simulink model "fuzzy_pid_control2"  (Simulink 8.7)
settings: Solver=VariableStepAuto  StartTime=0.0  StopTime=35  RelTol=1e-3
values from neighbouring files (symbols this model uses):
  M = 2.5    [matlab_11.mat]
  miu = 4.6    [matlab_11.mat]
undefined symbols (not defined in the file): name1, name2, name3
settings Model: Creator=Administrator  LastModifiedBy=Administrator
settings DataIOCC: LimitDataPoints=off  SaveFormat=Dataset
settings DebuggingCC: UnderspecifiedInitializationDetection=Simplified  MergeDetectMultiDrivingBlocksExec=error
settings HardwareCC: ProdBitPerPointer=64  ProdLargestAtomicFloat=Float  ProdIntDivRoundTo=Zero  ProdEndianess=LittleEndian  ProdWordSize=64  ProdHWDeviceType=Intel->x86-64 (Windows64)
settings ModelReferenceCC: PropagateSignalLabelsOutOfModel=on
settings ConfigComp: CovModelRefEnable=off

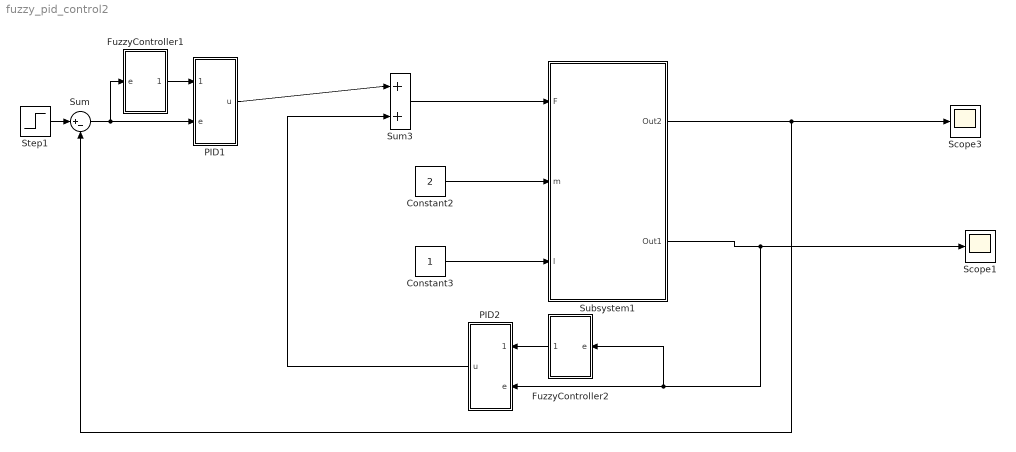
== system fuzzy_pid_control2 ==
  Constant2 : Constant  Value=2
  Constant3 : Constant
  FuzzyController1 : Subsystem
  FuzzyController2 : Subsystem
  PID1 : Subsystem
  PID2 : Subsystem
  Scope1 : Scope
  Scope3 : Scope
  Step1 : Step  Time=0  SampleTime=0
  Subsystem1 : Subsystem
  Sum : Sum  Inputs=|+-
  Sum3 : Sum  Inputs=|++
  wires:
  Step1/1 -> Sum/1
  Sum/1 -> PID1/2(e), FuzzyController1/1(e)
  Subsystem1/1(Out2) -> Scope3/1, Sum/2
  FuzzyController1/1(dPID) -> PID1/1(dPID)
  Constant2/1 -> Subsystem1/2(m)
  Constant3/1 -> Subsystem1/3(l)
  Sum3/1 -> Subsystem1/1(F)
  PID1/1(u) -> Sum3/1
  Subsystem1/2(Out1) -> FuzzyController2/1(e), PID2/2(e), Scope1/1
  PID2/1(u) -> Sum3/2
  FuzzyController2/1(dPID) -> PID2/1(dPID)

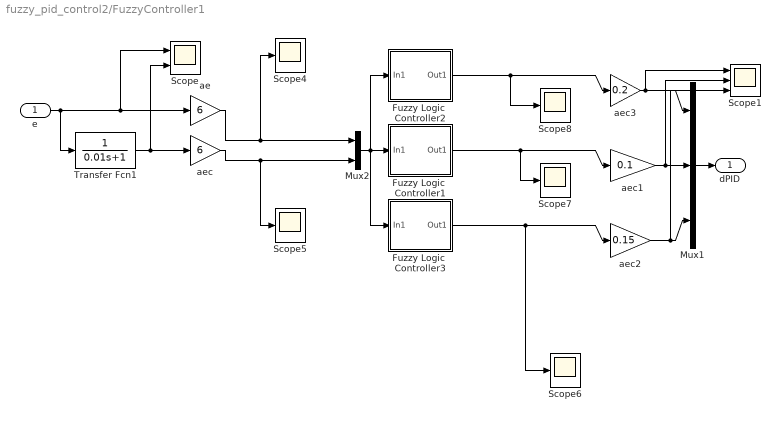
== system fuzzy_pid_control2/FuzzyController1 ==
  e : Inport
  Fuzzy Logic  Controller1 : Subsystem  AncestorBlock="fuzblock/Fuzzy Logic  Controller"  mask(FIS){fis=name3}
      mask prompts: fis "FIS File or Structure:"
      mask help: FIS
      mask init:
      | fis = fuzblockmask(gcb,fis);
      mask Help: web(['file:///' docroot '/toolbox/fuzzy/fuzzylogiccontroller.html']);
      mask Display: plot(0, -0.3, 6, -0.3, 0, 1.2, 6, 1.2, [0 6], [0 0], [1 2 3],[0 1 0],[2 3 4],[0 1 0],[3 4 5],[0 1 0])
  Fuzzy Logic  Controller2 : Subsystem  AncestorBlock="fuzblock/Fuzzy Logic  Controller"  mask(FIS){fis=name1}
      mask prompts: fis "FIS File or Structure:"
      mask help: FIS
      mask init:
      | fis = fuzblockmask(gcb,fis);
      mask Help: web(['file:///' docroot '/toolbox/fuzzy/fuzzylogiccontroller.html']);
      mask Display: plot(0, -0.3, 6, -0.3, 0, 1.2, 6, 1.2, [0 6], [0 0], [1 2 3],[0 1 0],[2 3 4],[0 1 0],[3 4 5],[0 1 0])
  Fuzzy Logic  Controller3 : Subsystem  AncestorBlock="fuzblock/Fuzzy Logic  Controller"  mask(FIS){fis=name2}
      mask prompts: fis "FIS File or Structure:"
      mask help: FIS
      mask init:
      | fis = fuzblockmask(gcb,fis);
      mask Help: web(['file:///' docroot '/toolbox/fuzzy/fuzzylogiccontroller.html']);
      mask Display: plot(0, -0.3, 6, -0.3, 0, 1.2, 6, 1.2, [0 6], [0 0], [1 2 3],[0 1 0],[2 3 4],[0 1 0],[3 4 5],[0 1 0])
  Mux1 : Mux  Inputs=3
  Mux2 : Mux  Inputs=2
  Scope : Scope  NumInputPorts=2
  Scope1 : Scope  NumInputPorts=3
  Scope{4..8} (5 alike) : Scope
  Transfer Fcn1 : TransferFcn  Denominator=[0.01 1]
  ae : Gain  Gain=6
  aec : Gain  Gain=6
  aec1 : Gain  Gain=0.1
  aec2 : Gain  Gain=0.15
  aec3 : Gain  Gain=0.2
  dPID : Outport
  wires:
  Fuzzy Logic  Controller2/1(Out1) -> aec3/1, Scope8/1
  Fuzzy Logic  Controller1/1(Out1) -> aec1/1, Scope7/1
  Fuzzy Logic  Controller3/1(Out1) -> aec2/1, Scope6/1
  e/1 -> Transfer Fcn1/1, ae/1, Scope/1
  Transfer Fcn1/1 -> aec/1, Scope/2
  ae/1 -> Mux2/1, Scope4/1
  aec/1 -> Mux2/2, Scope5/1
  Mux2/1 -> Fuzzy Logic  Controller1/1(In1), Fuzzy Logic  Controller3/1(In1), Fuzzy Logic  Controller2/1(In1)
  aec1/1 -> Mux1/2, Scope1/2
  aec2/1 -> Mux1/3, Scope1/3
  aec3/1 -> Mux1/1, Scope1/1
  Mux1/1 -> dPID/1

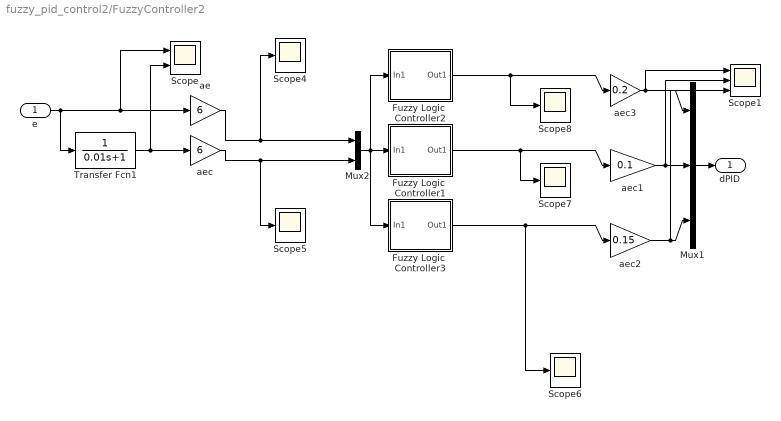
== system fuzzy_pid_control2/FuzzyController2 ==
  e : Inport
  Fuzzy Logic  Controller1 : Subsystem  AncestorBlock="fuzblock/Fuzzy Logic  Controller"  mask(FIS){fis=name3}
      mask prompts: fis "FIS File or Structure:"
      mask help: FIS
      mask init:
      | fis = fuzblockmask(gcb,fis);
      mask Help: web(['file:///' docroot '/toolbox/fuzzy/fuzzylogiccontroller.html']);
      mask Display: plot(0, -0.3, 6, -0.3, 0, 1.2, 6, 1.2, [0 6], [0 0], [1 2 3],[0 1 0],[2 3 4],[0 1 0],[3 4 5],[0 1 0])
  Fuzzy Logic  Controller2 : Subsystem  AncestorBlock="fuzblock/Fuzzy Logic  Controller"  mask(FIS){fis=name1}
      mask prompts: fis "FIS File or Structure:"
      mask help: FIS
      mask init:
      | fis = fuzblockmask(gcb,fis);
      mask Help: web(['file:///' docroot '/toolbox/fuzzy/fuzzylogiccontroller.html']);
      mask Display: plot(0, -0.3, 6, -0.3, 0, 1.2, 6, 1.2, [0 6], [0 0], [1 2 3],[0 1 0],[2 3 4],[0 1 0],[3 4 5],[0 1 0])
  Fuzzy Logic  Controller3 : Subsystem  AncestorBlock="fuzblock/Fuzzy Logic  Controller"  mask(FIS){fis=name2}
      mask prompts: fis "FIS File or Structure:"
      mask help: FIS
      mask init:
      | fis = fuzblockmask(gcb,fis);
      mask Help: web(['file:///' docroot '/toolbox/fuzzy/fuzzylogiccontroller.html']);
      mask Display: plot(0, -0.3, 6, -0.3, 0, 1.2, 6, 1.2, [0 6], [0 0], [1 2 3],[0 1 0],[2 3 4],[0 1 0],[3 4 5],[0 1 0])
  Mux1 : Mux  Inputs=3
  Mux2 : Mux  Inputs=2
  Scope : Scope  NumInputPorts=2
  Scope1 : Scope  NumInputPorts=3
  Scope{4..8} (5 alike) : Scope
  Transfer Fcn1 : TransferFcn  Denominator=[0.01 1]
  ae : Gain  Gain=6
  aec : Gain  Gain=6
  aec1 : Gain  Gain=0.1
  aec2 : Gain  Gain=0.15
  aec3 : Gain  Gain=0.2
  dPID : Outport
  wires:
  Fuzzy Logic  Controller2/1(Out1) -> aec3/1, Scope8/1
  Fuzzy Logic  Controller1/1(Out1) -> aec1/1, Scope7/1
  Fuzzy Logic  Controller3/1(Out1) -> aec2/1, Scope6/1
  e/1 -> Transfer Fcn1/1, ae/1, Scope/1
  Transfer Fcn1/1 -> aec/1, Scope/2
  ae/1 -> Mux2/1, Scope4/1
  aec/1 -> Mux2/2, Scope5/1
  Mux2/1 -> Fuzzy Logic  Controller1/1(In1), Fuzzy Logic  Controller3/1(In1), Fuzzy Logic  Controller2/1(In1)
  aec1/1 -> Mux1/2, Scope1/2
  aec2/1 -> Mux1/3, Scope1/3
  aec3/1 -> Mux1/1, Scope1/1
  Mux1/1 -> dPID/1

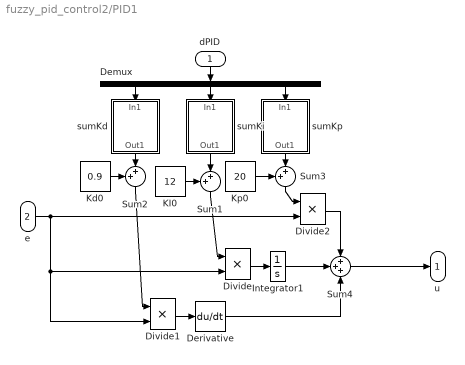
== system fuzzy_pid_control2/PID1 ==
  dPID : Inport
  e : Inport  Port=2
  Demux : Demux  Outputs=3
  Derivative : Derivative
  Divide : Product  Inputs=**
  Divide1 : Product  Inputs=**
  Divide2 : Product  Inputs=**
  Integrator1 : Integrator
  KI0 : Constant  Value=12
  Kd0 : Constant  Value=0.9
  Kp0 : Constant  Value=20
  Sum1 : Sum  Inputs=++|
  Sum2 : Sum  Inputs=++|
  Sum3 : Sum  Inputs=++|
  Sum4 : Sum  Inputs=+++
  sumKd : Subsystem
  sumKi : Subsystem
  sumKp : Subsystem
  u : Outport
  wires:
  Sum3/1 -> Divide2/1
  Sum2/1 -> Divide1/1
  Kp0/1 -> Sum3/1
  Kd0/1 -> Sum2/1
  KI0/1 -> Sum1/1
  Sum1/1 -> Divide/1
  e/1 -> Divide2/2, Divide/2, Divide1/2
  Divide2/1 -> Sum4/1
  Divide/1 -> Integrator1/1
  Divide1/1 -> Derivative/1
  Sum4/1 -> u/1
  dPID/1 -> Demux/1
  Demux/3 -> sumKp/1(In1)
  Demux/2 -> sumKi/1(In1)
  Demux/1 -> sumKd/1(In1)
  Integrator1/1 -> Sum4/2
  Derivative/1 -> Sum4/3
  sumKp/1(Out1) -> Sum3/2
  sumKi/1(Out1) -> Sum1/2
  sumKd/1(Out1) -> Sum2/2

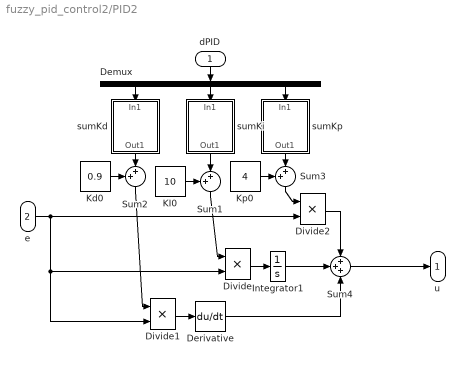
== system fuzzy_pid_control2/PID2 ==
  dPID : Inport
  e : Inport  Port=2
  Demux : Demux  Outputs=3
  Derivative : Derivative
  Divide : Product  Inputs=**
  Divide1 : Product  Inputs=**
  Divide2 : Product  Inputs=**
  Integrator1 : Integrator
  KI0 : Constant  Value=10
  Kd0 : Constant  Value=0.9
  Kp0 : Constant  Value=4
  Sum1 : Sum  Inputs=++|
  Sum2 : Sum  Inputs=++|
  Sum3 : Sum  Inputs=++|
  Sum4 : Sum  Inputs=+++
  sumKd : Subsystem
  sumKi : Subsystem
  sumKp : Subsystem
  u : Outport
  wires:
  Sum3/1 -> Divide2/1
  Sum2/1 -> Divide1/1
  Kp0/1 -> Sum3/1
  Kd0/1 -> Sum2/1
  KI0/1 -> Sum1/1
  Sum1/1 -> Divide/1
  e/1 -> Divide2/2, Divide/2, Divide1/2
  Divide2/1 -> Sum4/1
  Divide/1 -> Integrator1/1
  Divide1/1 -> Derivative/1
  Sum4/1 -> u/1
  dPID/1 -> Demux/1
  Demux/3 -> sumKp/1(In1)
  Demux/2 -> sumKi/1(In1)
  Demux/1 -> sumKd/1(In1)
  Integrator1/1 -> Sum4/2
  Derivative/1 -> Sum4/3
  sumKp/1(Out1) -> Sum3/2
  sumKi/1(Out1) -> Sum1/2
  sumKd/1(Out1) -> Sum2/2

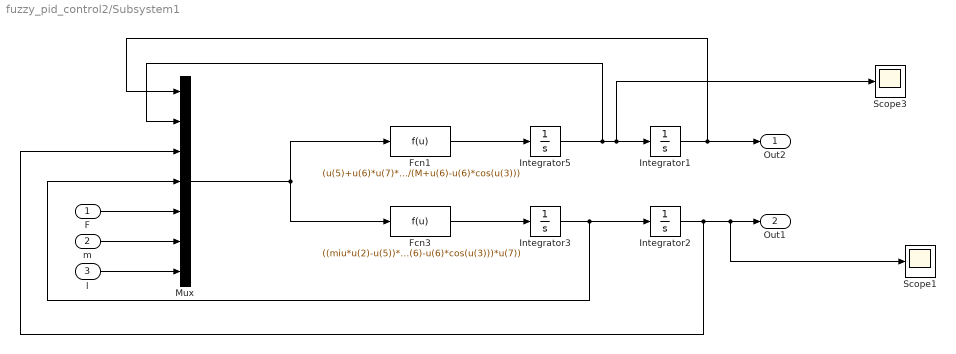
== system fuzzy_pid_control2/Subsystem1 ==
  F : Inport
  m : Inport  Port=2
  l : Inport  Port=3
  Fcn1 : Fcn  Expr=(u(5)+u(6)*u(7)*u(4)*u(4)*sin(u(3))+9.8*u(6)*sin(u(3))-miu*u(2))/(M+u(6)-u(6)*cos(u(3)))
  Fcn3 : Fcn  Expr=((miu*u(2)-u(5))*u(7)*cos(u(3))-(u(7)*u(7)*u(4)*u(4)+9.8*u(7)*9.8)*u(6)*sin(u(3))*cos(u(3))-(M+u(6))*9.8*sin(u(3)))/((M+u(6)-u(6)*cos(u(3)))*u(7))
  Integrator{1..3,5} (4 alike) : Integrator
  Mux : Mux  Inputs=7
  Scope1 : Scope
  Scope3 : Scope
  Out2 : Outport
  Out1 : Outport  Port=2
  wires:
  Integrator1/1 -> Out2/1, Mux/1
  l/1 -> Mux/7
  Fcn3/1 -> Integrator3/1
  F/1 -> Mux/5
  Integrator3/1 -> Mux/4, Integrator2/1
  Integrator5/1 -> Mux/2, Scope3/1, Integrator1/1
  m/1 -> Mux/6
  Mux/1 -> Fcn3/1, Fcn1/1
  Fcn1/1 -> Integrator5/1
  Integrator2/1 -> Scope1/1, Out1/1, Mux/3

== system fuzzy_pid_control2/FuzzyController1/Fuzzy Logic  Controller1 ==
  In1 : Inport
  FIS S-function : S-Function  FunctionName=sffis  Parameters=fis  SFunctionModules=sfsup  SFunctionDeploymentMode=off  EnableBusSupport=off
  Out1 : Outport
  wires:
  FIS S-function/1 -> Out1/1
  In1/1 -> FIS S-function/1

== system fuzzy_pid_control2/FuzzyController1/Fuzzy Logic  Controller2 ==
  In1 : Inport
  FIS S-function : S-Function  FunctionName=sffis  Parameters=fis  SFunctionModules=sfsup  SFunctionDeploymentMode=off  EnableBusSupport=off
  Out1 : Outport
  wires:
  In1/1 -> FIS S-function/1
  FIS S-function/1 -> Out1/1

== system fuzzy_pid_control2/FuzzyController1/Fuzzy Logic  Controller3 ==
  In1 : Inport
  FIS S-function : S-Function  FunctionName=sffis  Parameters=fis  SFunctionModules=sfsup  SFunctionDeploymentMode=off  EnableBusSupport=off
  Out1 : Outport
  wires:
  In1/1 -> FIS S-function/1
  FIS S-function/1 -> Out1/1

== system fuzzy_pid_control2/FuzzyController2/Fuzzy Logic  Controller1 ==
  In1 : Inport
  FIS S-function : S-Function  FunctionName=sffis  Parameters=fis  SFunctionModules=sfsup  SFunctionDeploymentMode=off  EnableBusSupport=off
  Out1 : Outport
  wires:
  FIS S-function/1 -> Out1/1
  In1/1 -> FIS S-function/1

== system fuzzy_pid_control2/FuzzyController2/Fuzzy Logic  Controller2 ==
  In1 : Inport
  FIS S-function : S-Function  FunctionName=sffis  Parameters=fis  SFunctionModules=sfsup  SFunctionDeploymentMode=off  EnableBusSupport=off
  Out1 : Outport
  wires:
  In1/1 -> FIS S-function/1
  FIS S-function/1 -> Out1/1

== system fuzzy_pid_control2/FuzzyController2/Fuzzy Logic  Controller3 ==
  In1 : Inport
  FIS S-function : S-Function  FunctionName=sffis  Parameters=fis  SFunctionModules=sfsup  SFunctionDeploymentMode=off  EnableBusSupport=off
  Out1 : Outport
  wires:
  In1/1 -> FIS S-function/1
  FIS S-function/1 -> Out1/1

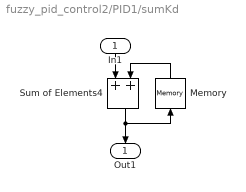
== system fuzzy_pid_control2/PID1/sumKd ==
  In1 : Inport
  Memory : Memory  InheritSampleTime=on
  Sum of Elements4 : Sum  SampleTime=0.001
  Out1 : Outport
  wires:
  Sum of Elements4/1 -> Out1/1, Memory/1
  Memory/1 -> Sum of Elements4/2
  In1/1 -> Sum of Elements4/1

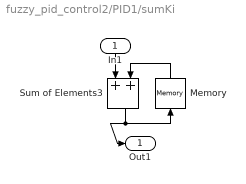
== system fuzzy_pid_control2/PID1/sumKi ==
  In1 : Inport
  Memory : Memory  InheritSampleTime=on
  Sum of Elements3 : Sum  SampleTime=0.001
  Out1 : Outport
  wires:
  Sum of Elements3/1 -> Out1/1, Memory/1
  Memory/1 -> Sum of Elements3/2
  In1/1 -> Sum of Elements3/1

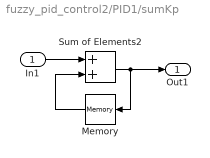
== system fuzzy_pid_control2/PID1/sumKp ==
  In1 : Inport
  Memory : Memory  InheritSampleTime=on
  Sum of Elements2 : Sum  SampleTime=0.001
  Out1 : Outport
  wires:
  In1/1 -> Sum of Elements2/1
  Memory/1 -> Sum of Elements2/2
  Sum of Elements2/1 -> Out1/1, Memory/1

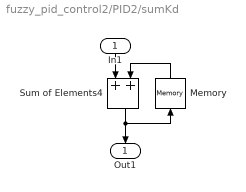
== system fuzzy_pid_control2/PID2/sumKd ==
  In1 : Inport
  Memory : Memory  InheritSampleTime=on
  Sum of Elements4 : Sum  SampleTime=0.001
  Out1 : Outport
  wires:
  Sum of Elements4/1 -> Out1/1, Memory/1
  Memory/1 -> Sum of Elements4/2
  In1/1 -> Sum of Elements4/1

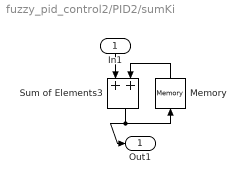
== system fuzzy_pid_control2/PID2/sumKi ==
  In1 : Inport
  Memory : Memory  InheritSampleTime=on
  Sum of Elements3 : Sum  SampleTime=0.001
  Out1 : Outport
  wires:
  Sum of Elements3/1 -> Out1/1, Memory/1
  Memory/1 -> Sum of Elements3/2
  In1/1 -> Sum of Elements3/1

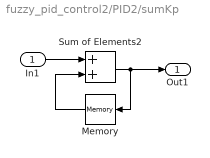
== system fuzzy_pid_control2/PID2/sumKp ==
  In1 : Inport
  Memory : Memory  InheritSampleTime=on
  Sum of Elements2 : Sum  SampleTime=0.001
  Out1 : Outport
  wires:
  In1/1 -> Sum of Elements2/1
  Memory/1 -> Sum of Elements2/2
  Sum of Elements2/1 -> Out1/1, Memory/1
